simulink model "SAMM_Dynamic"  (R2025b)
settings: Solver=ode45  StartTime=0.0  StopTime=4.0  MaxStep=0.01  RelTol=1e-4
settings Model: Creator=HP  LastModifiedBy=HP

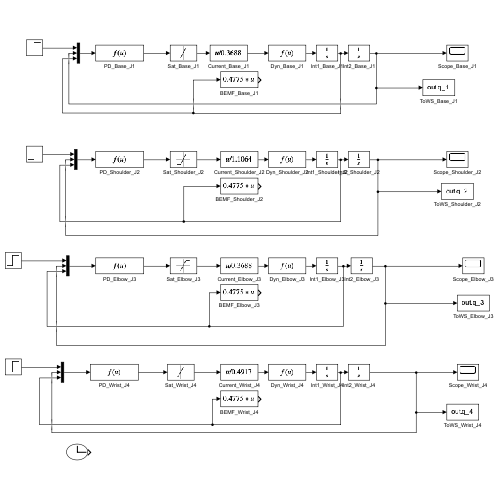
[thumbnail: Simulink's stored preview of the top-level diagram]
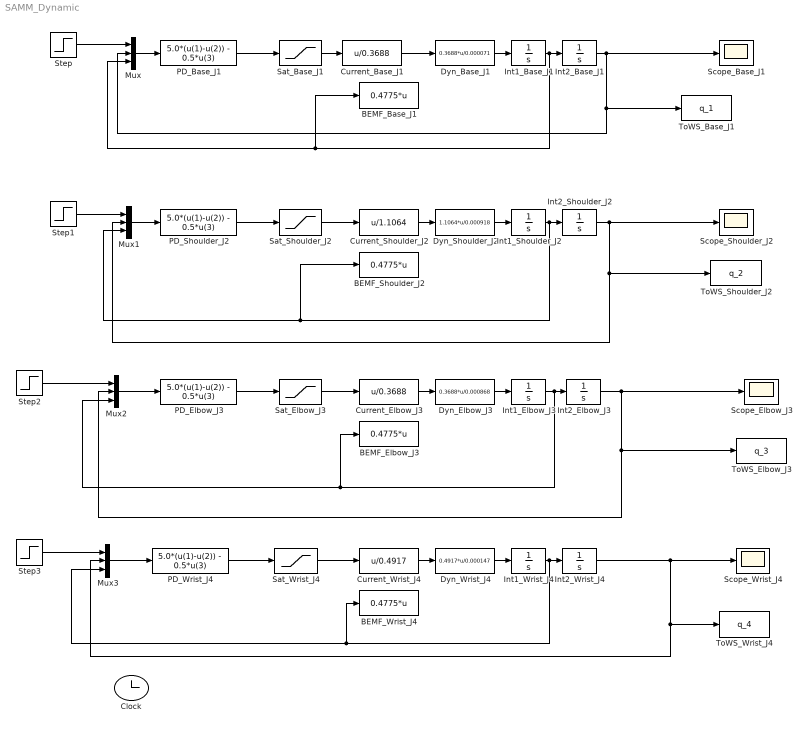
== system SAMM_Dynamic ==
  BEMF_Base_J1 : Fcn  Expr=0.4775*u
  BEMF_Elbow_J3 : Fcn  Expr=0.4775*u
  BEMF_Shoulder_J2 : Fcn  Expr=0.4775*u
  BEMF_Wrist_J4 : Fcn  Expr=0.4775*u
  Clock : Clock
  Current_Base_J1 : Fcn  Expr=u/0.3688
  Current_Elbow_J3 : Fcn  Expr=u/0.3688
  Current_Shoulder_J2 : Fcn  Expr=u/1.1064
  Current_Wrist_J4 : Fcn  Expr=u/0.4917
  Dyn_Base_J1 : Fcn  Expr=0.3688*u/0.000071
  Dyn_Elbow_J3 : Fcn  Expr=0.3688*u/0.000868
  Dyn_Shoulder_J2 : Fcn  Expr=1.1064*u/0.000918
  Dyn_Wrist_J4 : Fcn  Expr=0.4917*u/0.000147
  Int1_Base_J1 : Integrator
  Int1_Elbow_J3 : Integrator
  Int1_Shoulder_J2 : Integrator
  Int1_Wrist_J4 : Integrator
  Int2_Base_J1 : Integrator
  Int2_Elbow_J3 : Integrator
  Int2_Shoulder_J2 : Integrator
  Int2_Wrist_J4 : Integrator
  Mux{,1..3} (4 alike) : Mux  Inputs=3
  PD_Base_J1 : Fcn  Expr=5.0*(u(1)-u(2)) - 0.5*u(3)
  PD_Elbow_J3 : Fcn  Expr=5.0*(u(1)-u(2)) - 0.5*u(3)
  PD_Shoulder_J2 : Fcn  Expr=5.0*(u(1)-u(2)) - 0.5*u(3)
  PD_Wrist_J4 : Fcn  Expr=5.0*(u(1)-u(2)) - 0.5*u(3)
  Sat_Base_J1 : Saturate  UpperLimit=6  LowerLimit=-6
  Sat_Elbow_J3 : Saturate  UpperLimit=0.922  LowerLimit=-0.922
  Sat_Shoulder_J2 : Saturate  UpperLimit=2.766  LowerLimit=-2.766
  Sat_Wrist_J4 : Saturate  UpperLimit=0.177  LowerLimit=-0.177
  Scope_Base_J1 : Scope
      settings: ActiveDisplayYMinimum=-0.12499999881919385  ActiveDisplayYMaximum=1.1249999893727449
  Scope_Elbow_J3 : Scope
      settings: ActiveDisplayYMinimum=-0.12499999999999278  ActiveDisplayYMaximum=1.1249999999999354
  Scope_Shoulder_J2 : Scope
      settings: ActiveDisplayYMinimum=-0.12499999999999296  ActiveDisplayYMaximum=1.1249999999999369
  Scope_Wrist_J4 : Scope
      settings: ActiveDisplayYMinimum=-0.1249999999999888  ActiveDisplayYMaximum=1.1249999999998994
  Step{,1..3} (4 alike) : Step  SampleTime=0
  ToWS_Base_J1 : ToWorkspace  VariableName=q_1  SampleTime=-1
  ToWS_Elbow_J3 : ToWorkspace  VariableName=q_3  SampleTime=-1
  ToWS_Shoulder_J2 : ToWorkspace  VariableName=q_2  SampleTime=-1
  ToWS_Wrist_J4 : ToWorkspace  VariableName=q_4  SampleTime=-1
  wires:
  PD_Base_J1/1 -> Sat_Base_J1/1
  Sat_Base_J1/1 -> Current_Base_J1/1
  Current_Base_J1/1 -> Dyn_Base_J1/1
  Dyn_Base_J1/1 -> Int1_Base_J1/1
  Int1_Base_J1/1 -> Mux/3, BEMF_Base_J1/1, Int2_Base_J1/1
  Int2_Base_J1/1 -> Mux/2, ToWS_Base_J1/1, Scope_Base_J1/1
  Step/1 -> Mux/1
  Mux/1 -> PD_Base_J1/1
  Step1/1 -> Mux1/1
  Mux1/1 -> PD_Shoulder_J2/1
  PD_Shoulder_J2/1 -> Sat_Shoulder_J2/1
  Sat_Shoulder_J2/1 -> Current_Shoulder_J2/1
  Current_Shoulder_J2/1 -> Dyn_Shoulder_J2/1
  Dyn_Shoulder_J2/1 -> Int1_Shoulder_J2/1
  Int1_Shoulder_J2/1 -> BEMF_Shoulder_J2/1, Mux1/3, Int2_Shoulder_J2/1
  Int2_Shoulder_J2/1 -> ToWS_Shoulder_J2/1, Mux1/2, Scope_Shoulder_J2/1
  Mux3/1 -> PD_Wrist_J4/1
  Mux2/1 -> PD_Elbow_J3/1
  Step2/1 -> Mux2/1
  Step3/1 -> Mux3/1
  PD_Elbow_J3/1 -> Sat_Elbow_J3/1
  Sat_Elbow_J3/1 -> Current_Elbow_J3/1
  Current_Elbow_J3/1 -> Dyn_Elbow_J3/1
  Dyn_Elbow_J3/1 -> Int1_Elbow_J3/1
  Dyn_Wrist_J4/1 -> Int1_Wrist_J4/1
  Current_Wrist_J4/1 -> Dyn_Wrist_J4/1
  Sat_Wrist_J4/1 -> Current_Wrist_J4/1
  PD_Wrist_J4/1 -> Sat_Wrist_J4/1
  Int1_Elbow_J3/1 -> BEMF_Elbow_J3/1, Mux2/3, Int2_Elbow_J3/1
  Int2_Elbow_J3/1 -> Scope_Elbow_J3/1, ToWS_Elbow_J3/1, Mux2/2
  Int2_Wrist_J4/1 -> ToWS_Wrist_J4/1, Mux3/2, Scope_Wrist_J4/1
  Int1_Wrist_J4/1 -> Mux3/3, BEMF_Wrist_J4/1, Int2_Wrist_J4/1
